simulink model "tyre_model_v2"  (R2024b)
settings: Solver=FixedStepDiscrete  StartTime=0.0  StopTime=10.0  FixedStep=Ts  RelTol=1e-3
settings Model: Creator=marti  LastModifiedBy=marti

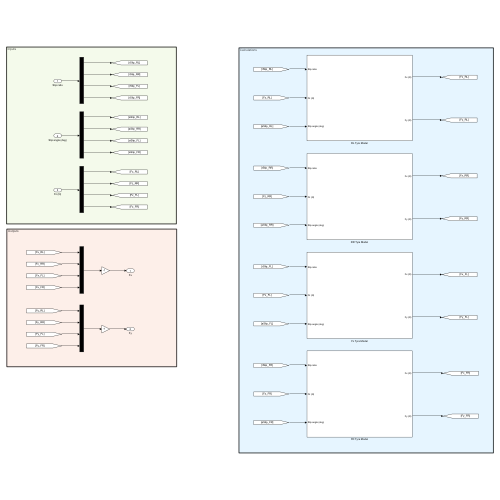
[thumbnail: Simulink's stored preview of the top-level diagram]
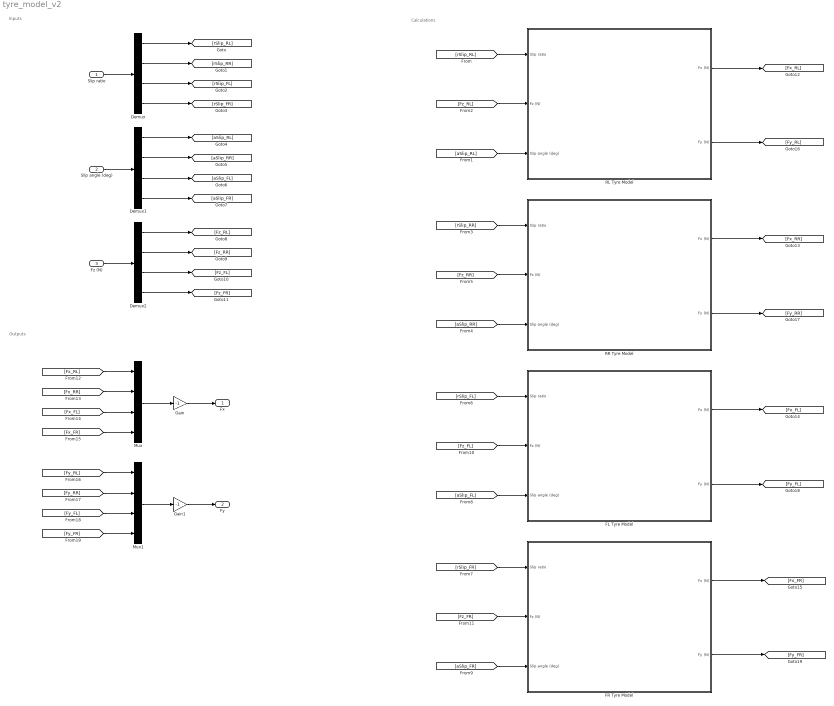
== system tyre_model_v2 ==
  note: Calculations
  note: Outputs
  note: Inputs
  Slip ratio : Inport
  Slip angle (deg) : Inport  Port=2
  Fz (N) : Inport  Port=3
  Demux : Demux
  Demux1 : Demux
  Demux2 : Demux
  FL Tyre Model : Subsystem
  FR Tyre Model : Subsystem
  Gain : Gain  Gain=-1
  Gain1 : Gain  Gain=-1
  Mux : Mux
  Mux1 : Mux
  RL Tyre Model : Subsystem
  RR Tyre Model : Subsystem
  Fx : Outport
  Fy : Outport  Port=2
  wires:
  Slip ratio/1 -> Demux/1
  Demux/1 -> [rSlip_RL]
  Demux/2 -> [rSlip_RR]
  Demux/3 -> [rSlip_FL]
  Demux/4 -> [rSlip_FR]
  Demux1/4 -> [aSlip_FR]
  Demux1/3 -> [aSlip_FL]
  Demux1/2 -> [aSlip_RR]
  Demux1/1 -> [aSlip_RL]
  Slip angle (deg)/1 -> Demux1/1
  Demux2/1 -> [Fz_RL]
  Demux2/2 -> [Fz_RR]
  Demux2/3 -> [Fz_FL]
  Demux2/4 -> [Fz_FR]
  Fz (N)/1 -> Demux2/1
  [rSlip_RL] -> RL Tyre Model/1(Slip ratio)
  [Fz_RL] -> RL Tyre Model/2(Fz (N))
  [aSlip_RL] -> RL Tyre Model/3(Slip angle (deg))
  [rSlip_RR] -> RR Tyre Model/1(Slip ratio)
  [aSlip_RR] -> RR Tyre Model/3(Slip angle (deg))
  [Fz_RR] -> RR Tyre Model/2(Fz (N))
  [rSlip_FL] -> FL Tyre Model/1(Slip ratio)
  [rSlip_FR] -> FR Tyre Model/1(Slip ratio)
  [aSlip_FL] -> FL Tyre Model/3(Slip angle (deg))
  [aSlip_FR] -> FR Tyre Model/3(Slip angle (deg))
  [Fz_FL] -> FL Tyre Model/2(Fz (N))
  [Fz_FR] -> FR Tyre Model/2(Fz (N))
  RL Tyre Model/1(Fx (N)) -> [Fx_RL]
  RR Tyre Model/1(Fx (N)) -> [Fx_RR]
  FL Tyre Model/1(Fx (N)) -> [Fx_FL]
  FR Tyre Model/1(Fx (N)) -> [Fx_FR]
  RL Tyre Model/2(Fy (N)) -> [Fy_RL]
  RR Tyre Model/2(Fy (N)) -> [Fy_RR]
  FL Tyre Model/2(Fy (N)) -> [Fy_FL]
  FR Tyre Model/2(Fy (N)) -> [Fy_FR]
  [Fx_RL] -> Mux/1
  [Fx_RR] -> Mux/2
  [Fx_FL] -> Mux/3
  [Fx_FR] -> Mux/4
  Mux/1 -> Gain/1
  Mux1/1 -> Gain1/1
  [Fy_FR] -> Mux1/4
  [Fy_FL] -> Mux1/3
  [Fy_RR] -> Mux1/2
  [Fy_RL] -> Mux1/1
  Gain/1 -> Fx/1
  Gain1/1 -> Fy/1

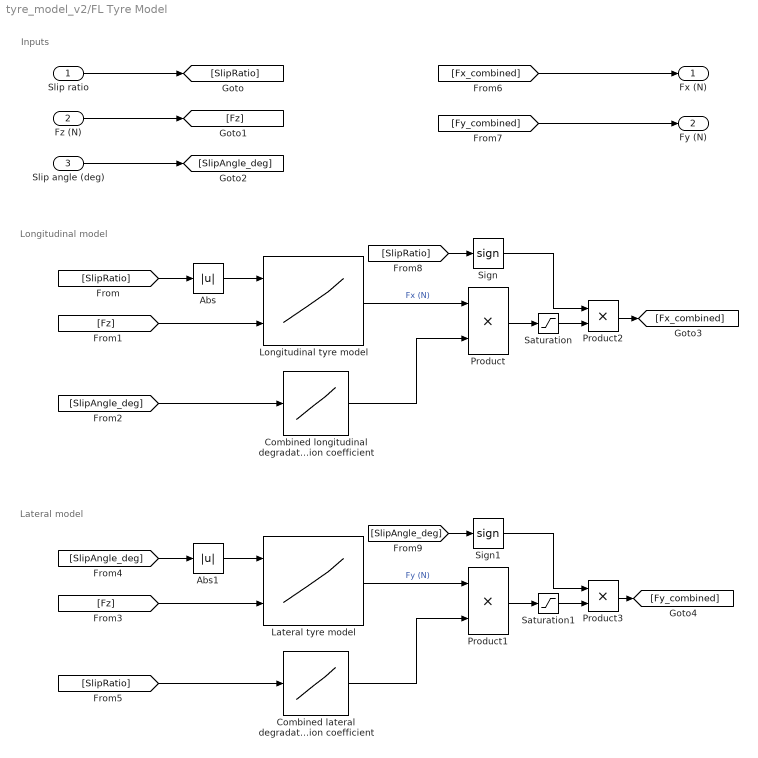
== system tyre_model_v2/FL Tyre Model ==
  note: Inputs
  note: Lateral model
  note: Longitudinal model
  Slip ratio : Inport
  Fz (N) : Inport  Port=2
  Slip angle (deg) : Inport  Port=3
  Abs : Abs  SaturateOnIntegerOverflow=off
  Abs1 : Abs  SaturateOnIntegerOverflow=off
  Combined lateral degradation coefficient : Lookup_n-D  NumberOfTableDimensions=1  BreakpointsForDimension1=[0 0.05 0.1 0.2]  Table=[1 0.95 0.8 0.4]  InternalRulePriority=Speed  RndMeth=Simplest
  Combined longitudinal degradation coefficient : Lookup_n-D  NumberOfTableDimensions=1  BreakpointsForDimension1=[0 3 6 10]  Table=[1 0.95 0.8 0.4]  InternalRulePriority=Speed  RndMeth=Simplest
  Lateral tyre model : Lookup_n-D  BreakpointsForDimension1=[0;2.5;5;7.5;10;12.5;15]  BreakpointsForDimension2=[200;400;650;1100;1450;1600]  Table=[0 0 0 0 0 0;160 180 715 715 1240 1300;260 280 1030 1040 1840 1900;340 345 1250 1275 2440 2500;380 380 1350 1360 2600 2630;370 375 1400 1410 2575 2600;370 390 1380 1390 2525 2550]  InternalRulePriority=Speed  RndMeth=Simplest
      settings: InputPortMap=u0,u1
  Longitudinal tyre model : Lookup_n-D  BreakpointsForDimension1=[0;0.025000000000000001;0.050000000000000003;0.074999999999999997;0.10000000000000001;0.125;0.14999999999999999;0.17499999999999999;0.20000000000000001]  BreakpointsForDimension2=[150;250;600;700;1050;1150;1500]  Table=[0 0 0 0 0 0 0;160 180 715 715 1240 1300 1520;260 280 1030 1040 1840 1900 2400;340 345 1250 1275 2440 2500 3050;380 380 1350 1360 2600 2630 3300;370 375 1400 1410 2575 2600 3400;370 390 1380 1390 2525 2550 3350;360 370 1370 1385 2400 2430 3300;350 360 1350 1370 2300 2330 3100]  InternalRulePriority=Speed  RndMeth=Simplest
      settings: InputPortMap=u0,u1
  Product{,1..3} (4 alike) : Product
  Saturation : Saturate  UpperLimit=4000  LowerLimit=0
  Saturation1 : Saturate  UpperLimit=4000  LowerLimit=0
  Sign : Signum
  Sign1 : Signum
  Fx (N) : Outport
  Fy (N) : Outport  Port=2
  wires:
  Saturation/1 -> Product2/2
  [SlipAngle_deg] -> Sign1/1
  Abs1/1 -> Lateral tyre model/1
  Product/1 -> Saturation/1
  [SlipRatio] -> Combined lateral degradation coefficient/1
  Abs/1 -> Longitudinal tyre model/1
  Product1/1 -> Saturation1/1
  [Fy_combined] -> Fy (N)/1
  Sign1/1 -> Product3/1
  Saturation1/1 -> Product3/2
  Longitudinal tyre model/1 -> Product/1  "Fx (N)"
  [SlipAngle_deg] -> Abs1/1
  [Fz] -> Longitudinal tyre model/2
  [SlipAngle_deg] -> Combined longitudinal degradation coefficient/1
  Combined longitudinal degradation coefficient/1 -> Product/2
  Lateral tyre model/1 -> Product1/1  "Fy (N)"
  [Fz] -> Lateral tyre model/2
  Product2/1 -> [Fx_combined]
  Sign/1 -> Product2/1
  Fz (N)/1 -> [Fz]
  [Fx_combined] -> Fx (N)/1
  [SlipRatio] -> Abs/1
  [SlipRatio] -> Sign/1
  Slip ratio/1 -> [SlipRatio]
  Combined lateral degradation coefficient/1 -> Product1/2
  Product3/1 -> [Fy_combined]
  Slip angle (deg)/1 -> [SlipAngle_deg]

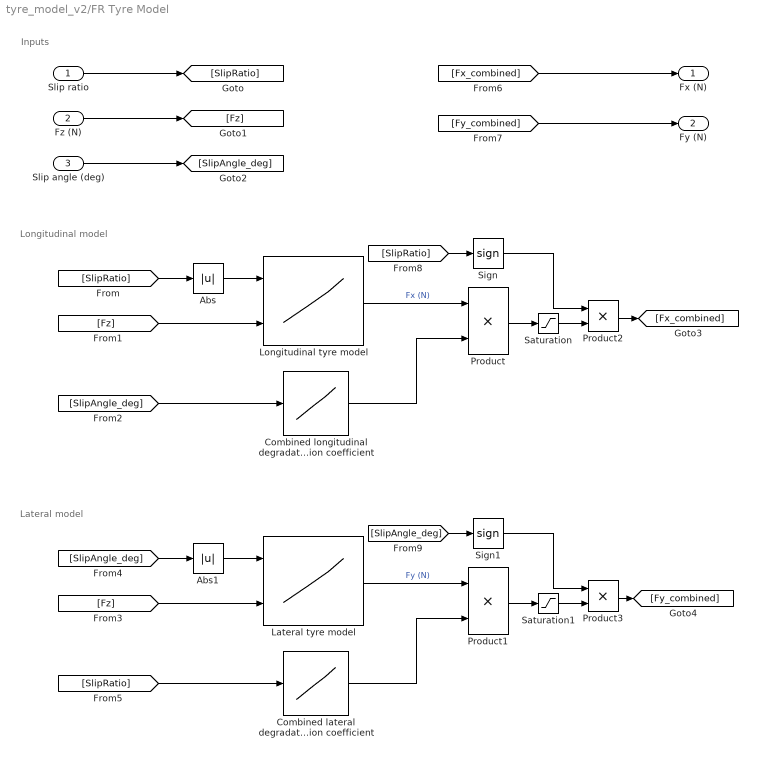
== system tyre_model_v2/FR Tyre Model ==
  note: Inputs
  note: Lateral model
  note: Longitudinal model
  Slip ratio : Inport
  Fz (N) : Inport  Port=2
  Slip angle (deg) : Inport  Port=3
  Abs : Abs  SaturateOnIntegerOverflow=off
  Abs1 : Abs  SaturateOnIntegerOverflow=off
  Combined lateral degradation coefficient : Lookup_n-D  NumberOfTableDimensions=1  BreakpointsForDimension1=[0 0.05 0.1 0.2]  Table=[1 0.95 0.8 0.4]  InternalRulePriority=Speed  RndMeth=Simplest
  Combined longitudinal degradation coefficient : Lookup_n-D  NumberOfTableDimensions=1  BreakpointsForDimension1=[0 3 6 10]  Table=[1 0.95 0.8 0.4]  InternalRulePriority=Speed  RndMeth=Simplest
  Lateral tyre model : Lookup_n-D  BreakpointsForDimension1=[0;2.5;5;7.5;10;12.5;15]  BreakpointsForDimension2=[200;400;650;1100;1450;1600]  Table=[0 0 0 0 0 0;160 180 715 715 1240 1300;260 280 1030 1040 1840 1900;340 345 1250 1275 2440 2500;380 380 1350 1360 2600 2630;370 375 1400 1410 2575 2600;370 390 1380 1390 2525 2550]  InternalRulePriority=Speed  RndMeth=Simplest
      settings: InputPortMap=u0,u1
  Longitudinal tyre model : Lookup_n-D  BreakpointsForDimension1=[0;0.025000000000000001;0.050000000000000003;0.074999999999999997;0.10000000000000001;0.125;0.14999999999999999;0.17499999999999999;0.20000000000000001]  BreakpointsForDimension2=[150;250;600;700;1050;1150;1500]  Table=[0 0 0 0 0 0 0;160 180 715 715 1240 1300 1520;260 280 1030 1040 1840 1900 2400;340 345 1250 1275 2440 2500 3050;380 380 1350 1360 2600 2630 3300;370 375 1400 1410 2575 2600 3400;370 390 1380 1390 2525 2550 3350;360 370 1370 1385 2400 2430 3300;350 360 1350 1370 2300 2330 3100]  InternalRulePriority=Speed  RndMeth=Simplest
      settings: InputPortMap=u0,u1
  Product{,1..3} (4 alike) : Product
  Saturation : Saturate  UpperLimit=4000  LowerLimit=0
  Saturation1 : Saturate  UpperLimit=4000  LowerLimit=0
  Sign : Signum
  Sign1 : Signum
  Fx (N) : Outport
  Fy (N) : Outport  Port=2
  wires:
  Saturation/1 -> Product2/2
  [SlipAngle_deg] -> Sign1/1
  Abs1/1 -> Lateral tyre model/1
  Product/1 -> Saturation/1
  [SlipRatio] -> Combined lateral degradation coefficient/1
  Abs/1 -> Longitudinal tyre model/1
  Product1/1 -> Saturation1/1
  [Fy_combined] -> Fy (N)/1
  Sign1/1 -> Product3/1
  Saturation1/1 -> Product3/2
  Longitudinal tyre model/1 -> Product/1  "Fx (N)"
  [SlipAngle_deg] -> Abs1/1
  [Fz] -> Longitudinal tyre model/2
  [SlipAngle_deg] -> Combined longitudinal degradation coefficient/1
  Combined longitudinal degradation coefficient/1 -> Product/2
  Lateral tyre model/1 -> Product1/1  "Fy (N)"
  [Fz] -> Lateral tyre model/2
  Product2/1 -> [Fx_combined]
  Sign/1 -> Product2/1
  Fz (N)/1 -> [Fz]
  [Fx_combined] -> Fx (N)/1
  [SlipRatio] -> Abs/1
  [SlipRatio] -> Sign/1
  Slip ratio/1 -> [SlipRatio]
  Combined lateral degradation coefficient/1 -> Product1/2
  Product3/1 -> [Fy_combined]
  Slip angle (deg)/1 -> [SlipAngle_deg]

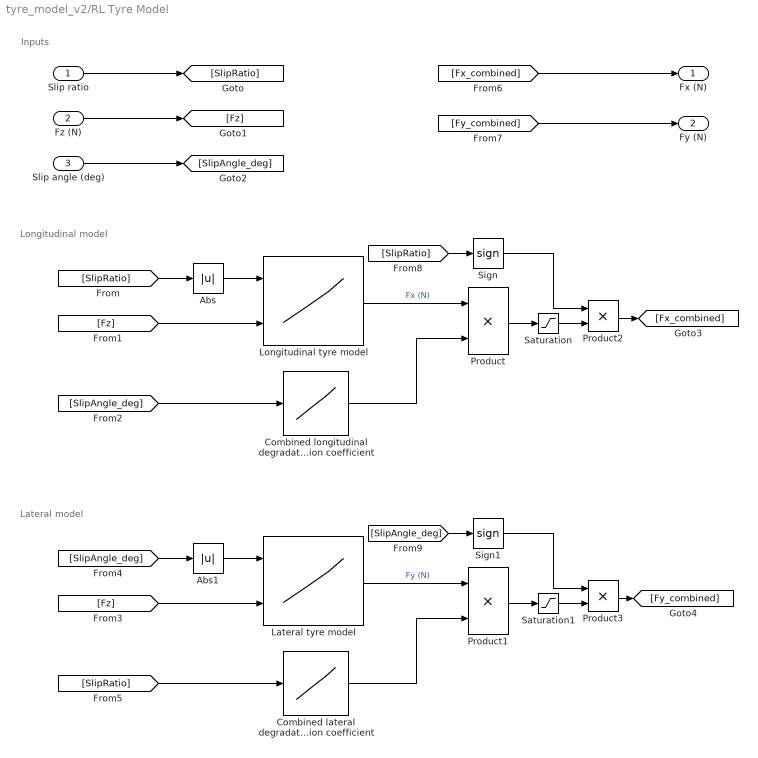
== system tyre_model_v2/RL Tyre Model ==
  note: Longitudinal model
  note: Inputs
  note: Lateral model
  Slip ratio : Inport
  Fz (N) : Inport  Port=2
  Slip angle (deg) : Inport  Port=3
  Abs : Abs  SaturateOnIntegerOverflow=off
  Abs1 : Abs  SaturateOnIntegerOverflow=off
  Combined lateral degradation coefficient : Lookup_n-D  NumberOfTableDimensions=1  BreakpointsForDimension1=[0 0.05 0.1 0.2]  Table=[1 0.95 0.8 0.4]  InternalRulePriority=Speed  RndMeth=Simplest
  Combined longitudinal degradation coefficient : Lookup_n-D  NumberOfTableDimensions=1  BreakpointsForDimension1=[0 3 6 10]  Table=[1 0.95 0.8 0.4]  InternalRulePriority=Speed  RndMeth=Simplest
  Lateral tyre model : Lookup_n-D  BreakpointsForDimension1=[0;2.5;5;7.5;10;12.5;15]  BreakpointsForDimension2=[200;400;650;1100;1450;1600]  Table=[0 0 0 0 0 0;160 180 715 715 1240 1300;260 280 1030 1040 1840 1900;340 345 1250 1275 2440 2500;380 380 1350 1360 2600 2630;370 375 1400 1410 2575 2600;370 390 1380 1390 2525 2550]  InternalRulePriority=Speed  RndMeth=Simplest
      settings: InputPortMap=u0,u1
  Longitudinal tyre model : Lookup_n-D  BreakpointsForDimension1=[0;0.025000000000000001;0.050000000000000003;0.074999999999999997;0.10000000000000001;0.125;0.14999999999999999;0.17499999999999999;0.20000000000000001]  BreakpointsForDimension2=[150;250;600;700;1050;1150;1500]  Table=[0 0 0 0 0 0 0;160 180 715 715 1240 1300 1520;260 280 1030 1040 1840 1900 2400;340 345 1250 1275 2440 2500 3050;380 380 1350 1360 2600 2630 3300;370 375 1400 1410 2575 2600 3400;370 390 1380 1390 2525 2550 3350;360 370 1370 1385 2400 2430 3300;350 360 1350 1370 2300 2330 3100]  InternalRulePriority=Speed  RndMeth=Simplest
      settings: InputPortMap=u0,u1
  Product{,1..3} (4 alike) : Product
  Saturation : Saturate  UpperLimit=4000  LowerLimit=0
  Saturation1 : Saturate  UpperLimit=4000  LowerLimit=0
  Sign : Signum
  Sign1 : Signum
  Fx (N) : Outport
  Fy (N) : Outport  Port=2
  wires:
  Abs1/1 -> Lateral tyre model/1
  Abs/1 -> Longitudinal tyre model/1
  Product3/1 -> [Fy_combined]
  Product1/1 -> Saturation1/1
  [SlipAngle_deg] -> Sign1/1
  Sign1/1 -> Product3/1
  Sign/1 -> Product2/1
  [SlipRatio] -> Sign/1
  Product/1 -> Saturation/1
  Product2/1 -> [Fx_combined]
  Lateral tyre model/1 -> Product1/1  "Fy (N)"
  Combined lateral degradation coefficient/1 -> Product1/2
  [Fx_combined] -> Fx (N)/1
  [SlipRatio] -> Combined lateral degradation coefficient/1
  [Fy_combined] -> Fy (N)/1
  [SlipAngle_deg] -> Abs1/1
  [Fz] -> Longitudinal tyre model/2
  [Fz] -> Lateral tyre model/2
  Fz (N)/1 -> [Fz]
  Longitudinal tyre model/1 -> Product/1  "Fx (N)"
  [SlipRatio] -> Abs/1
  Slip angle (deg)/1 -> [SlipAngle_deg]
  Combined longitudinal degradation coefficient/1 -> Product/2
  Slip ratio/1 -> [SlipRatio]
  [SlipAngle_deg] -> Combined longitudinal degradation coefficient/1
  Saturation/1 -> Product2/2
  Saturation1/1 -> Product3/2

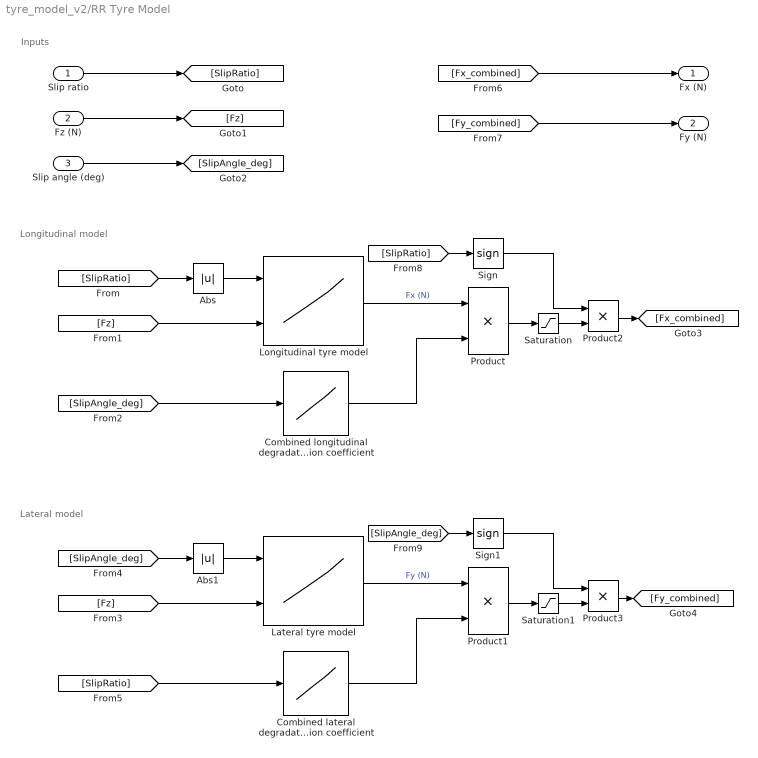
== system tyre_model_v2/RR Tyre Model ==
  note: Inputs
  note: Lateral model
  note: Longitudinal model
  Slip ratio : Inport
  Fz (N) : Inport  Port=2
  Slip angle (deg) : Inport  Port=3
  Abs : Abs  SaturateOnIntegerOverflow=off
  Abs1 : Abs  SaturateOnIntegerOverflow=off
  Combined lateral degradation coefficient : Lookup_n-D  NumberOfTableDimensions=1  BreakpointsForDimension1=[0 0.05 0.1 0.2]  Table=[1 0.95 0.8 0.4]  InternalRulePriority=Speed  RndMeth=Simplest
  Combined longitudinal degradation coefficient : Lookup_n-D  NumberOfTableDimensions=1  BreakpointsForDimension1=[0 3 6 10]  Table=[1 0.95 0.8 0.4]  InternalRulePriority=Speed  RndMeth=Simplest
  Lateral tyre model : Lookup_n-D  BreakpointsForDimension1=[0;2.5;5;7.5;10;12.5;15]  BreakpointsForDimension2=[200;400;650;1100;1450;1600]  Table=[0 0 0 0 0 0;160 180 715 715 1240 1300;260 280 1030 1040 1840 1900;340 345 1250 1275 2440 2500;380 380 1350 1360 2600 2630;370 375 1400 1410 2575 2600;370 390 1380 1390 2525 2550]  InternalRulePriority=Speed  RndMeth=Simplest
      settings: InputPortMap=u0,u1
  Longitudinal tyre model : Lookup_n-D  BreakpointsForDimension1=[0;0.025000000000000001;0.050000000000000003;0.074999999999999997;0.10000000000000001;0.125;0.14999999999999999;0.17499999999999999;0.20000000000000001]  BreakpointsForDimension2=[150;250;600;700;1050;1150;1500]  Table=[0 0 0 0 0 0 0;160 180 715 715 1240 1300 1520;260 280 1030 1040 1840 1900 2400;340 345 1250 1275 2440 2500 3050;380 380 1350 1360 2600 2630 3300;370 375 1400 1410 2575 2600 3400;370 390 1380 1390 2525 2550 3350;360 370 1370 1385 2400 2430 3300;350 360 1350 1370 2300 2330 3100]  InternalRulePriority=Speed  RndMeth=Simplest
      settings: InputPortMap=u0,u1
  Product{,1..3} (4 alike) : Product
  Saturation : Saturate  UpperLimit=4000  LowerLimit=0
  Saturation1 : Saturate  UpperLimit=4000  LowerLimit=0
  Sign : Signum
  Sign1 : Signum
  Fx (N) : Outport
  Fy (N) : Outport  Port=2
  wires:
  Saturation/1 -> Product2/2
  [SlipAngle_deg] -> Sign1/1
  Abs1/1 -> Lateral tyre model/1
  Product/1 -> Saturation/1
  [SlipRatio] -> Combined lateral degradation coefficient/1
  Abs/1 -> Longitudinal tyre model/1
  Product1/1 -> Saturation1/1
  [Fy_combined] -> Fy (N)/1
  Sign1/1 -> Product3/1
  Saturation1/1 -> Product3/2
  Longitudinal tyre model/1 -> Product/1  "Fx (N)"
  [SlipAngle_deg] -> Abs1/1
  [Fz] -> Longitudinal tyre model/2
  [SlipAngle_deg] -> Combined longitudinal degradation coefficient/1
  Combined longitudinal degradation coefficient/1 -> Product/2
  Lateral tyre model/1 -> Product1/1  "Fy (N)"
  [Fz] -> Lateral tyre model/2
  Product2/1 -> [Fx_combined]
  Sign/1 -> Product2/1
  Fz (N)/1 -> [Fz]
  [Fx_combined] -> Fx (N)/1
  [SlipRatio] -> Abs/1
  [SlipRatio] -> Sign/1
  Slip ratio/1 -> [SlipRatio]
  Combined lateral degradation coefficient/1 -> Product1/2
  Product3/1 -> [Fy_combined]
  Slip angle (deg)/1 -> [SlipAngle_deg]
